simulink model "PenObs"  (R2019b)
settings: Solver=VariableStepAuto  StartTime=0.0  StopTime=10.0  RelTol=1e-3
settings Model: Creator=aarij  LastModifiedBy=aarij

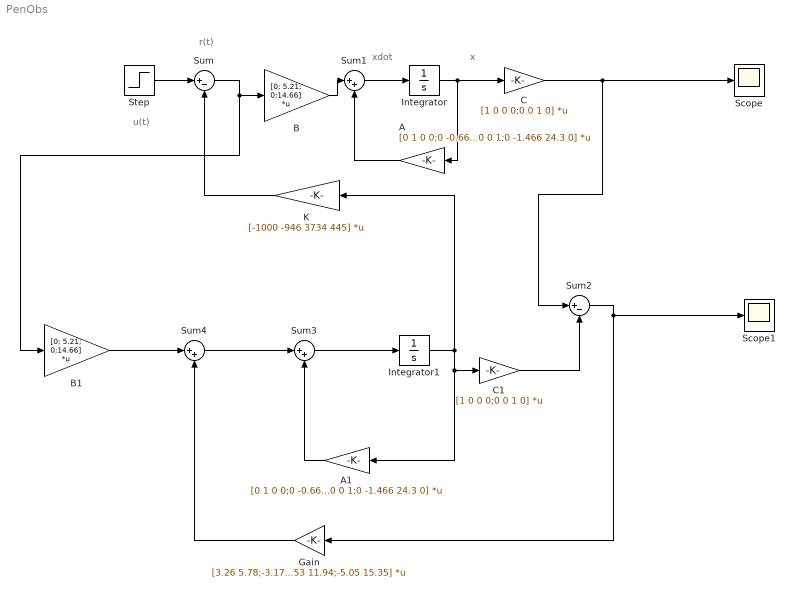
== system PenObs ==
  note: u(t)
  note: x
  note: xdot
  note: r(t)
  A : Gain  Gain=[0 1 0 0;0 -0.661 1.265 0; 0 0 0 1;0 -1.466 24.3 0]  Multiplication=Matrix(K*u)
  A1 : Gain  Gain=[0 1 0 0;0 -0.661 1.265 0; 0 0 0 1;0 -1.466 24.3 0]  Multiplication=Matrix(K*u)
  B : Gain  Gain=[0; 5.21; 0;14.66]  Multiplication=Matrix(K*u) (u vector)
  B1 : Gain  Gain=[0; 5.21; 0;14.66]  Multiplication=Matrix(K*u)
  C : Gain  Gain=[1 0 0 0;0 0 1 0]  Multiplication=Matrix(K*u)
  C1 : Gain  Gain=[1 0 0 0;0 0 1 0]  Multiplication=Matrix(K*u)
  Gain : Gain  Gain=[3.26 5.78;-3.176 -4.35;5.53 11.94;-5.05 15.35]  Multiplication=Matrix(K*u) (u vector)
  Integrator : Integrator
  Integrator1 : Integrator
  K : Gain  Gain=[-1000 -946 3734 445]  Multiplication=Matrix(K*u) (u vector)
  Scope : Scope
  Scope1 : Scope
  Step : Step  Time=0  SampleTime=0
  Sum : Sum  Inputs=|+-
  Sum1 : Sum  Inputs=|++
  Sum2 : Sum  Inputs=|+-
  Sum3 : Sum  Inputs=|++
  Sum4 : Sum  Inputs=|++
  wires:
  Step/1 -> Sum/1
  B/1 -> Sum1/1
  Sum/1 -> B1/1, B/1
  Integrator/1 -> A/1, C/1
  Sum1/1 -> Integrator/1
  A/1 -> Sum1/2
  K/1 -> Sum/2
  C/1 -> Sum2/1, Scope/1
  A1/1 -> Sum3/2
  B1/1 -> Sum4/1
  Gain/1 -> Sum4/2
  Sum4/1 -> Sum3/1
  Sum3/1 -> Integrator1/1
  Integrator1/1 -> K/1, A1/1, C1/1
  C1/1 -> Sum2/2
  Sum2/1 -> Gain/1, Scope1/1
